simulink model "simulink_carro"  (R2017a)
settings: Solver=VariableStepAuto  StartTime=0.0  StopTime=50  RelTol=1e-3
values from neighbouring files (symbols this model uses):
  Area = 4    [script_carro.m]
  Cd = 0.29    [script_carro.m]
  Cr = 0.01    [script_carro.m]
  den = [5 -3]    [script_carro.m]
  m = 1626    [script_carro.m]
  num = 5000*[300 -260]    [script_carro.m]
  rho = 1.23    [script_carro.m]
  ts = 0.01    [script_carro.m]
libraries: simulink x1
settings Model: Creator=mozelli  LastModifiedBy=Italo

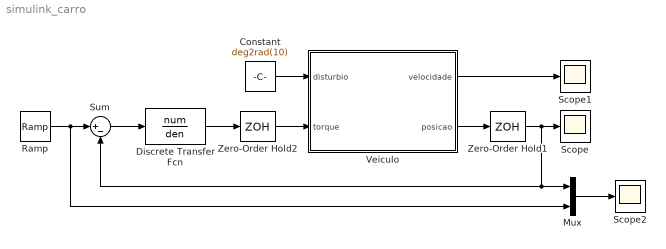
== system simulink_carro ==
  Constant : Constant  Value=deg2rad(10)
  Discrete Transfer Fcn : DiscreteTransferFcn  Numerator=num  Denominator=den
  Mux : Mux  Inputs=2
  Ramp : simulink/Sources/Ramp  slope=20  start=0  X0=0
  Scope : Scope
  Scope1 : Scope
  Scope2 : Scope
  Sum : Sum  Inputs=|+-
  Veiculo : Subsystem
      mask Display: image('honda.jpeg');
  Zero-Order Hold1 : ZeroOrderHold  SampleTime=ts
  Zero-Order Hold2 : ZeroOrderHold  SampleTime=ts
  wires:
  Constant/1 -> Veiculo/1(disturbio)
  Ramp/1 -> Mux/2, Sum/1
  Discrete Transfer Fcn/1 -> Zero-Order Hold2/1
  Veiculo/1(velocidade) -> Scope1/1
  Veiculo/2(posicao) -> Zero-Order Hold1/1
  Zero-Order Hold1/1 -> Mux/1, Sum/2, Scope/1
  Zero-Order Hold2/1 -> Veiculo/2(torque)
  Sum/1 -> Discrete Transfer Fcn/1
  Mux/1 -> Scope2/1

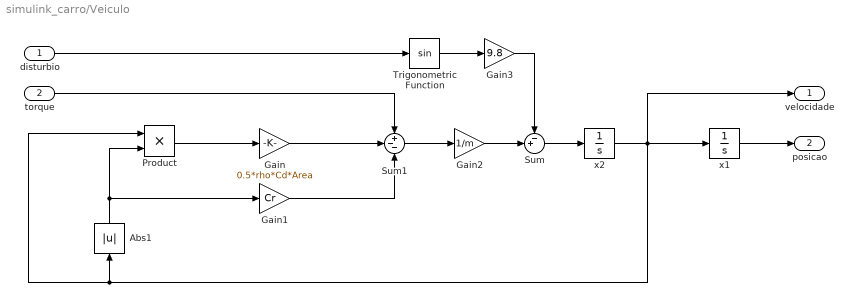
== system simulink_carro/Veiculo ==
  disturbio : Inport
  torque : Inport  Port=2
  Abs1 : Abs
  Gain : Gain  Gain=0.5*rho*Cd*Area
  Gain1 : Gain  Gain=Cr
  Gain2 : Gain  Gain=1/m
  Gain3 : Gain  Gain=9.8
  Product : Product
  Sum : Sum  Inputs=-+|
  Sum1 : Sum  Inputs=+--
  Trigonometric Function : Trigonometry
  x1 : Integrator  InitialCondition=2
  x2 : Integrator  InitialCondition=1
  velocidade : Outport
  posicao : Outport  Port=2
  wires:
  Product/1 -> Gain/1
  x1/1 -> posicao/1
  Gain1/1 -> Sum1/3
  Sum1/1 -> Gain2/1
  Abs1/1 -> Gain1/1, Product/2
  x2/1 -> velocidade/1, x1/1, Abs1/1, Product/1
  torque/1 -> Sum1/1
  Gain/1 -> Sum1/2
  Gain2/1 -> Sum/2
  disturbio/1 -> Trigonometric Function/1
  Trigonometric Function/1 -> Gain3/1
  Gain3/1 -> Sum/1
  Sum/1 -> x2/1
